simulink model "prova_appello1_sim"  (R2024a)
settings: Solver=VariableStepAuto  StartTime=0.0  StopTime=10.0  RelTol=1e-3
values from neighbouring files (symbols this model uses):
  A = [-2 8;0 -10]    [prova_appello_1.m]
  B = [2 2]'    [prova_appello_1.m]
undefined symbols (not defined in the file or in its folder): K1
settings Model: Creator=stefa  LastModifiedBy=stefa

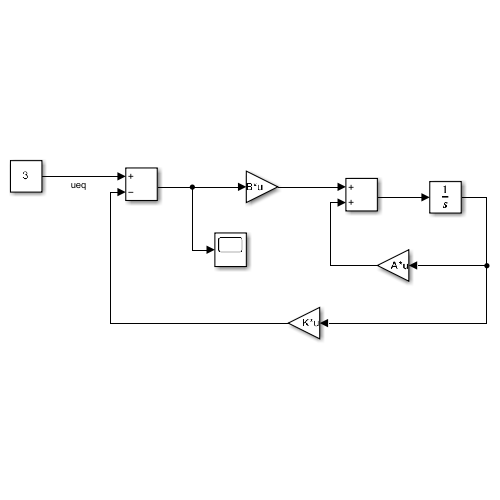
[thumbnail: Simulink's stored preview of the top-level diagram]
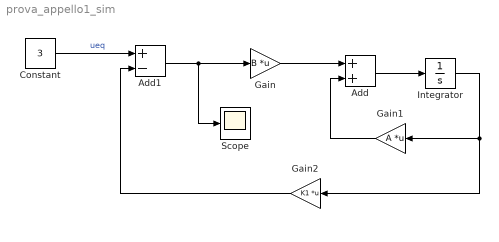
== system prova_appello1_sim ==
  Add : Sum
  Add1 : Sum  Inputs=+-
  Constant : Constant  Value=3
  Gain : Gain  Gain=B  Multiplication=Matrix(K*u)
  Gain1 : Gain  Gain=A  Multiplication=Matrix(K*u)
  Gain2 : Gain  Gain=K1  Multiplication=Matrix(K*u)
  Integrator : Integrator
  Scope : Scope
  wires:
  Integrator/1 -> Gain2/1, Gain1/1
  Gain1/1 -> Add/2
  Add/1 -> Integrator/1
  Gain/1 -> Add/1
  Add1/1 -> Scope/1, Gain/1
  Constant/1 -> Add1/1  "ueq"
  Gain2/1 -> Add1/2
